simulink subsystem "singleTrackDynF"  (R2021a)
settings: Solver=VariableStepAuto  StartTime=0.0  StopTime=10.0  RelTol=1e-3
model mask{leftORright=left track, m=0, trackwidth=0, trackgap=0, mu=0.5, K=0.2, r=0.3, l=1}
  mask prompts: leftORright "left or right track?"; m "vehicle mass"; trackwidth "track width"; trackgap "track latral gap"; mu "soil coefficient, mu"; K "soil unit length, K"; r "track drive wheel radius, r"; l "track length"
values from neighbouring files (symbols this model uses):
  K = 0.2    [hybridforce.m]    (also in trackedforce.m; trackforce.m)
  l = 2    [hybridforce.m]    (also in trackedforce.m; trackforce.m)
  m = 3e3    (= 3000)    [solveequilibrium.m]    (also in sspeverifyoptim.m; trackforce.m)
  mu = 0.5    [hybridforce.m]    (also in tireforce.m = 0.55; trackedforce.m; trackforce.m)
  r = 0.3    [hybridforce.m]    (also in trackedforce.m; trackforce.m)
undefined symbols (not defined in the file or in its folder): x_mesh, y_mesh
settings Model: Creator=polonium  LastModifiedBy=polonium

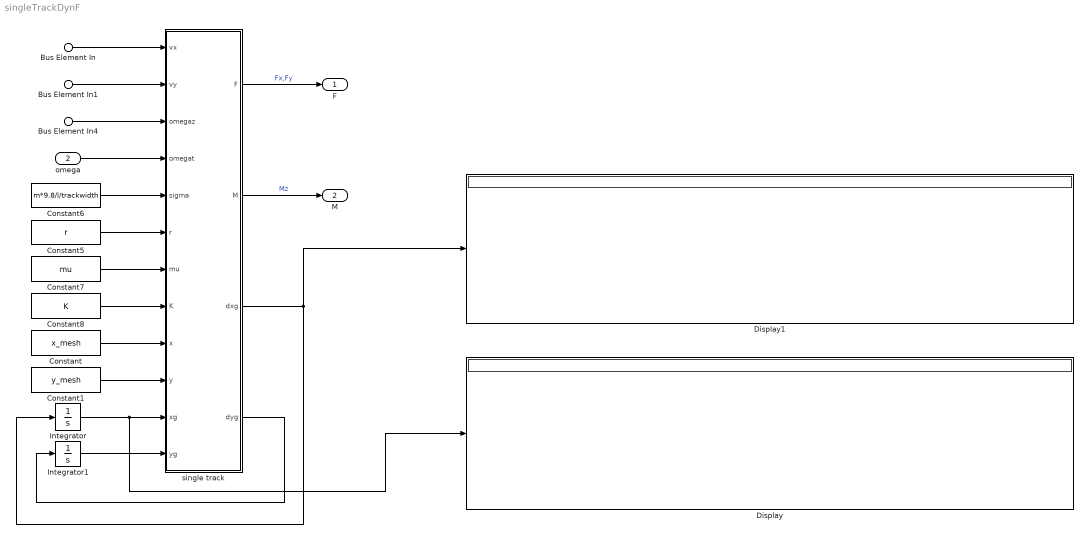
== system singleTrackDynF ==
  Bus Element In : Inport  PortName=vel  Element=vx
  Bus Element In1 : Inport  PortName=vel  Element=vy
  Bus Element In4 : Inport  PortName=vel  Element=omegaz
  omega : Inport  Port=2
  Constant : Constant  Value=x_mesh
  Constant1 : Constant  Value=y_mesh
  Constant5 : Constant  Value=r
  Constant6 : Constant  Value=m*9.8/l/trackwidth
  Constant7 : Constant  Value=mu
  Constant8 : Constant  Value=K
  Display : Display
  Display1 : Display
  Integrator : Integrator  InitialCondition=x_mesh
  Integrator1 : Integrator  InitialCondition=y_mesh
  single track : MATLAB Function  TreatAsAtomicUnit=on
  F : Outport
  M : Outport  Port=2
  wires:
  Bus Element In1/1 -> single track/2(vy)
  Constant8/1 -> single track/8(K)
  Constant6/1 -> single track/5(sigma)
  Constant5/1 -> single track/6(r)
  Constant7/1 -> single track/7(mu)
  Constant1/1 -> single track/10(y)
  Bus Element In/1 -> single track/1(vx)
  Bus Element In4/1 -> single track/3(omegaz)
  omega/1 -> single track/4(omegat)
  Constant/1 -> single track/9(x)
  Integrator1/1 -> single track/12(yg)
  single track/4(dyg) -> Integrator1/1
  single track/3(dxg) -> Display1/1, Integrator/1
  single track/1(F) -> F/1  "Fx,Fy"
  Integrator/1 -> Display/1, single track/11(xg)
  single track/2(M) -> M/1  "Mz"

== matlab function singleTrackDynF/single track ==
  data: vx input; F output; vy input; omegaz input; omegat input; sigma input; r input; mu input; K input; x input; y input; xg input; yg input; M output; dxg output; dyg output
function [F,M,dxg,dyg] = fcn(vx,vy,omegaz,omegat,sigma,r,mu,K,x,y,xg,yg)

[Fx,Fy,Mz,dxg,dyg] = dynamicTrackForce(vx,vy,omegaz,omegat,sigma,r,mu,K,x,y,xg,yg);

% MATLAB uses SAE coordinate

F = [Fx -Fy];

M = -Mz;

end
